simulink model "simu2"  (R2022b)
settings: Solver=VariableStepAuto  StartTime=0.0  StopTime=30  RelTol=1e-3
values from neighbouring files (symbols this model uses):
  c = 2    [matlab.mat]
  d = 4    [matlab.mat]
  k1 = 1    [matlab.mat]
settings Model: Creator=paola  LastModifiedBy=paola

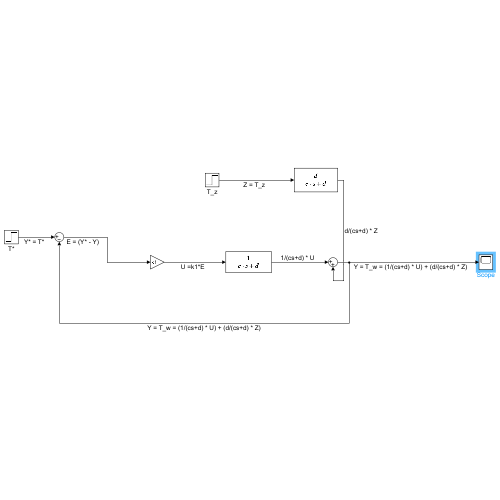
[thumbnail: Simulink's stored preview of the top-level diagram]
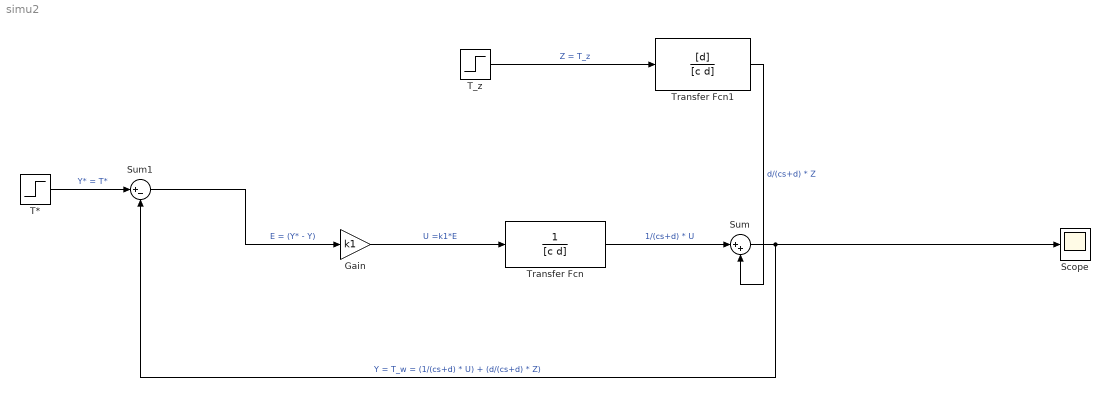
== system simu2 ==
  Gain : Gain  Gain=k1
  Scope : Scope
  Sum : Sum  Inputs=|++
  Sum1 : Sum  Inputs=|+-
  T* : Step  Time=2  SampleTime=0
  T_z : Step  Time=3  After=0  SampleTime=0
  Transfer Fcn : TransferFcn  Denominator=[c d]
  Transfer Fcn1 : TransferFcn  Numerator=[d]  Denominator=[c d]
  wires:
  Gain/1 -> Transfer Fcn/1  "U =k1*E"
  T_z/1 -> Transfer Fcn1/1  "Z = T_z"
  Sum/1 -> Sum1/2, Scope/1  "Y = T_w = (1/(cs+d) * U) + (d/(cs+d) * Z)"
  Transfer Fcn1/1 -> Sum/2  "d/(cs+d) * Z"
  Transfer Fcn/1 -> Sum/1  "1/(cs+d) * U"
  T*/1 -> Sum1/1  "Y* = T*"
  Sum1/1 -> Gain/1  "E = (Y* - Y)"
